simulink model "sumdiff_ec"  (Simulink 8.3)
settings: Solver=FixedStepDiscrete  StartTime=0.0  StopTime=inf  RelTol=1e-3
PostLoadFcn:
  | setsysloc(bdroot);
libraries: idelinkdemoslib x1, demo_controls x1
settings Model: Creator=The MathWorks Inc.  LastModifiedBy=gxnuhuang
settings SolverCC: PositivePriorityOrder=on
settings DataIOCC: SaveOutput=off  SignalLogging=off  SaveTime=off
settings OptimizationCC: ExpressionDepthLimit=2147483647  InitFltsAndDblsToZero=on  OptimizeModelRefInitCode=on  LifeSpan=1
settings DebuggingCC: SignalResolutionControl=TryResolveAllWithWarning  ParameterPrecisionLossMsg=none  FcnCallInpInsideContextMsg=UseLocalSettings
settings HardwareCC: ProdLargestAtomicInteger=Long  ProdLargestAtomicFloat=Double  ProdIntDivRoundTo=Zero  ProdEndianess=LittleEndian  ProdHWDeviceType=ARMCortex
settings RTWCC: SystemTargetFile=idelink_ert.tlc  GenerateMakefile=off  TemplateMakefile=none  Description=IDE Link ERT  GenerateReport=on  ProcessScript=idelink_ert_make_rtw_hook  IncludeHyperlinkInReport=on  LaunchReport=on
settings CodeAppCC: IgnoreCustomStorageClasses=off
settings ERTFactory: TargetFcnLib=ansi_tfl_table_tmw.mat  GenFloatMathFcnCalls=NOT IN USE  TargetLangStandard=C89/C90 (ANSI)  CodeReplacementLibrary=None  UtilityFuncGeneration=Auto  ERTMultiwordTypeDef=System defined  ERTMultiwordLength=256  MultiwordLength=2048  GenerateFullHeader=on  GenerateSampleERTMain=off  GenerateTestInterfaces=off  ModelReferenceCompliant=on  ParMdlRefBuildCompliant=off  CompOptLevelCompliant=off  ConcurrentExecutionCompliant=on  IncludeMdlTerminateFcn=on  GeneratePreprocessorConditionals=Disable all  CombineOutputUpdateFcns=on  CombineSignalStateStructs=off  SuppressErrorStatus=off  ERTFirstTimeCompliant=on  IncludeFileDelimiter=Auto  ERTCustomFileBanners=on  SupportAbsoluteTime=on  LogVarNameModifier=rt_  MatFileLogging=off  MultiInstanceERTCode=off  CodeInterfacePackaging=Nonreusable function  SupportNonFinite=on  SupportComplex=on  PurelyIntegerCode=off  SupportContinuousTime=off  SupportNonInlinedSFcns=off  SupportVariableSizeSignals=off  EnableShiftOperators=on  ParenthesesLevel=Nominal  MATLABClassNameForMDSCustomization=linkfoundation.pjtgenerator.IdelinkCustomization  ModelStepFunctionPrototypeControlCompliant=on  CPPClassGenCompliant=off  AutosarCompliant=off  GRTInterface=off  GenerateAllocFcn=off  GenerateASAP2=off  ExtMode=off  ExtModeTransport=0  ExtModeStaticAlloc=off  ExtModeStaticAllocSize=1000000  ExtModeTesting=off  ExtModeMexFile=ext_comm  ExtModeIntrfLevel=Level1  InlinedParameterPlacement=Hierarchical  TargetOS=BareBoardExample  MultiInstanceErrorCode=Error  RateGroupingCode=on  RootIOFormat=Individual arguments  RTWCAPISignals=off  RTWCAPIParams=off  RTWCAPIStates=off  RTWCAPIRootIO=off  ERTSrcFileBannerTemplate=ert_code_template.cgt  ERTHdrFileBannerTemplate=ert_code_template.cgt  ERTDataSrcFileTemplate=ert_code_template.cgt  ERTDataHdrFileTemplate=ert_code_template.cgt  ERTCustomFileTemplate=example_file_process.tlc  EnableDataOwnership=off  SignalDisplayLevel=10  ParamTuneLevel=10  GlobalDataDefinition=Auto  DataDefinitionFile=global.c  GlobalDataReference=Auto  ERTFilePackagingFormat=Modular  DataReferenceFile=global.h  PreserveExpressionOrder=off  PreserveIfCondition=off  ConvertIfToSwitch=off  PreserveExternInFcnDecls=on  SuppressUnreachableDefaultCases=off  IndentStyle=K&R  IndentSize=2  EnableUserReplacementTypes=off  MemSecPackage=--- None ---  MemSecDataConstants=Default  MemSecDataIO=Default  MemSecDataInternal=Default  MemSecDataParameters=Default  MemSecFuncInitTerm=Default  MemSecFuncExecute=Default  MemSecFuncSharedUtil=Default  AdaptorName=Eclipse  exportIDEObj=on  ideObjName=IDE_Objhzq  oldideObjName=IDE_Objhzq  ideObjTimeout=10  oldideObjTimeout=10  ideObjBuildTimeout=1000  oldideObjBuildTimeout=1000  TargetPrefTimeStamp=26-Aug-2014 09:31:00  ProfileGenCode=off  profileBy=Tasks  ProfileNumSamples=100  InlineDSPBlks=off  projectOptions=Custom  debugCompilerOptions="-g -D\"_DEBUG\""  releaseCompilerOptions=-O2  getCompilerOptions=off  resetCompilerOptions=off  debugLinkerOptions=-lm  releaseLinkerOptions=-lm  customLinkerOptions=-lm  linkerOptionsStr=-lm  getLinkerOptions=off  resetLinkerOptions=off  systemStackSize=131072  systemHeapSize=512  buildFormat=Project  buildAction=Build_and_execute  overrunNotificationMethod=Print_message  overrunNotificationFcn=myfunction  oldoverrunNotificationFcn=myfunction  configurePIL=off  configPILBlockAction=Create_PIL_block_build_and_download  TargetResourceManagerActiveTab=0  DiagnosticActions=warning
settings TargetHardwareResources: Description=Target Hardware Resources Component
settings MATStruct: cache=[]  boardType=BeagleBoard ARM  isSimulator=[0.0]  enableHSRTDX=[0.0]  versionNumber=2.9.1  enableDSPBIOSTab=[0.0]  RTOS=Linux  peripherals=[]  procName=4444  boardName=localhost  realtimesupport=off  tag=eclipseidetgtpref  deviceID=ARM Cortex-A8  subFamily=host  cpuClockRateMHz=[600.0]  codegenhookpoint=host  numRTOS=[2.0]  defaultSysStackSize=[131072.0]  isBuiltIn=[1.0]  numSections=[1.0]  numBanks=[1.0]  numCacheLvl=[0.0]  name=virtual_memory  contents=Code & Data  space=Internal  addr=[0.0]  size=[4096.0]  isremovable=[0.0]  iscontentsfixed=[0.0]  createHeap=[0.0]  heapSize=[0.0]  defineLabel=[0.0]  heapLabel=segment_name  label=None  timer=[]  timerprescaler=[]  description=Program code  codeObjectMem=virtual_memory  dataObjectMem=virtual_memory  section=[]  enable=off  schedulerType=Rate priority  schedulingMode=real-time  baseRatePriority=[40.0]  stackSize=[4096.0]  staticStackMemSegment=virtual_memory  dynamicStackMemSegment=virtual_memory  errId=[]

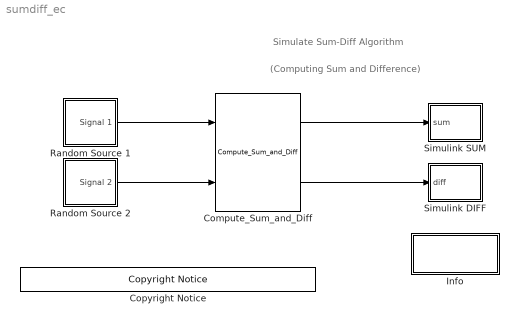
== system sumdiff_ec ==
  note: (Computing Sum and Difference)
  note: Simulate Sum-Diff Algorithm
  Compute_Sum_and_Diff : idelinkdemoslib/Compute_Sum_and_Diff
  Copyright Notice : demo_controls/Copyright Notice  year=2006  prod=idelink
  Info : Subsystem
      settings: OpenFcn=helpview(fullfile(idelinkdemodir('eclipseide'),'html','sumdiff_ec.html'));
      mask Help: helpview(fullfile(matlabroot,'toolbox','idelink','extensions','eclipseide','exlipseidedemos','html','publish_kworkflow.html'));
      mask Display: fprintf('Info');
  Random Source 1 : Subsystem
  Random Source 2 : Subsystem
  Simulink DIFF : Subsystem
  Simulink SUM : Subsystem
  wires:
  Random Source 1/1(Signal 1) -> Compute_Sum_and_Diff/1
  Random Source 2/1(Signal 2) -> Compute_Sum_and_Diff/2
  Compute_Sum_and_Diff/1 -> Simulink SUM/1(sum)
  Compute_Sum_and_Diff/2 -> Simulink DIFF/1(diff)

== system sumdiff_ec/Info ==

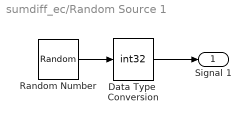
== system sumdiff_ec/Random Source 1 ==
  Data Type  Conversion : DataTypeConversion  OutDataTypeStr=int32  RndMeth=Nearest  SaturateOnIntegerOverflow=on
  Random Number : RandomNumber  Mean=zeros(16,1)  Variance=ones(16,1)  Seed=[1:16]'  SampleTime=1/1000  VectorParams1D=off
  Signal 1 : Outport
  wires:
  Random Number/1 -> Data Type  Conversion/1
  Data Type  Conversion/1 -> Signal 1/1

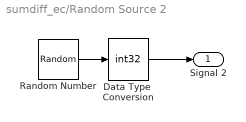
== system sumdiff_ec/Random Source 2 ==
  Data Type  Conversion : DataTypeConversion  OutDataTypeStr=int32  RndMeth=Nearest  SaturateOnIntegerOverflow=on
  Random Number : RandomNumber  Mean=zeros(16,1)  Variance=ones(16,1)  Seed=[2:17]'  SampleTime=1/1000  VectorParams1D=off
  Signal 2 : Outport
  wires:
  Random Number/1 -> Data Type  Conversion/1
  Data Type  Conversion/1 -> Signal 2/1

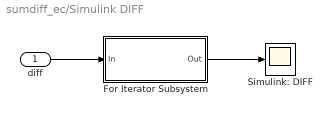
== system sumdiff_ec/Simulink DIFF ==
  diff : Inport
  For Iterator Subsystem : Subsystem  TreatAsAtomicUnit=on
  Simulink: DIFF : Scope
      settings: StartFcn=open_system(gcb);  TimeRange=0.016
  wires:
  diff/1 -> For Iterator Subsystem/1(In)
  For Iterator Subsystem/1(Out) -> Simulink: DIFF/1

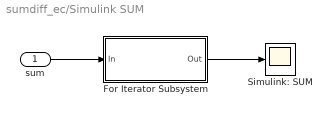
== system sumdiff_ec/Simulink SUM ==
  sum : Inport
  For Iterator Subsystem : Subsystem  TreatAsAtomicUnit=on
  Simulink: SUM : Scope
      settings: StartFcn=open_system(gcb);  TimeRange=0.016
  wires:
  sum/1 -> For Iterator Subsystem/1(In)
  For Iterator Subsystem/1(Out) -> Simulink: SUM/1

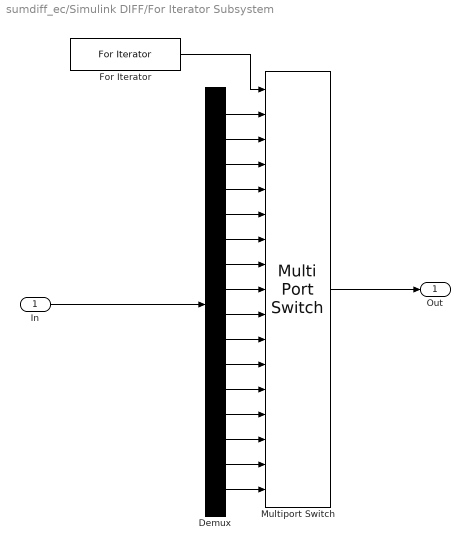
== system sumdiff_ec/Simulink DIFF/For Iterator Subsystem ==
  In : Inport
  Demux : Demux  Outputs=16
  For Iterator : ForIterator  ResetStates=reset  IterationLimit=16  IterationVariableDataType=int16
  Multiport Switch : MultiPortSwitch  Inputs=16
  Out : Outport
  wires:
  In/1 -> Demux/1
  Demux/16 -> Multiport Switch/17
  Demux/1 -> Multiport Switch/2
  Demux/2 -> Multiport Switch/3
  Demux/3 -> Multiport Switch/4
  Demux/4 -> Multiport Switch/5
  Demux/5 -> Multiport Switch/6
  Demux/6 -> Multiport Switch/7
  Demux/7 -> Multiport Switch/8
  Demux/8 -> Multiport Switch/9
  Demux/9 -> Multiport Switch/10
  Demux/10 -> Multiport Switch/11
  Demux/11 -> Multiport Switch/12
  Demux/12 -> Multiport Switch/13
  Demux/13 -> Multiport Switch/14
  Demux/14 -> Multiport Switch/15
  Demux/15 -> Multiport Switch/16
  Multiport Switch/1 -> Out/1
  For Iterator/1 -> Multiport Switch/1

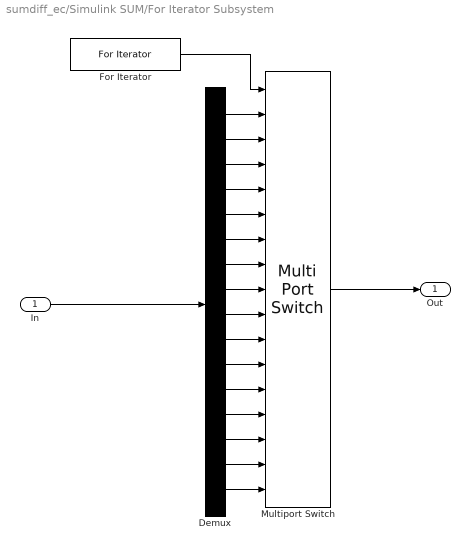
== system sumdiff_ec/Simulink SUM/For Iterator Subsystem ==
  In : Inport
  Demux : Demux  Outputs=16
  For Iterator : ForIterator  ResetStates=reset  IterationLimit=16  IterationVariableDataType=int16
  Multiport Switch : MultiPortSwitch  Inputs=16
  Out : Outport
  wires:
  In/1 -> Demux/1
  Demux/16 -> Multiport Switch/17
  Demux/1 -> Multiport Switch/2
  Demux/2 -> Multiport Switch/3
  Demux/3 -> Multiport Switch/4
  Demux/4 -> Multiport Switch/5
  Demux/5 -> Multiport Switch/6
  Demux/6 -> Multiport Switch/7
  Demux/7 -> Multiport Switch/8
  Demux/8 -> Multiport Switch/9
  Demux/9 -> Multiport Switch/10
  Demux/10 -> Multiport Switch/11
  Demux/11 -> Multiport Switch/12
  Demux/12 -> Multiport Switch/13
  Demux/13 -> Multiport Switch/14
  Demux/14 -> Multiport Switch/15
  Demux/15 -> Multiport Switch/16
  Multiport Switch/1 -> Out/1
  For Iterator/1 -> Multiport Switch/1
